simulink model "Example_2"  (R2020b)
settings: Solver=VariableStepAuto  StartTime=0.0  StopTime=0.001  RelTol=1e-3
libraries: fl_lib x10, nesl_utility x6, ee_lib x2
settings Model: Creator=zaliyazici  LastModifiedBy=zaliyazici

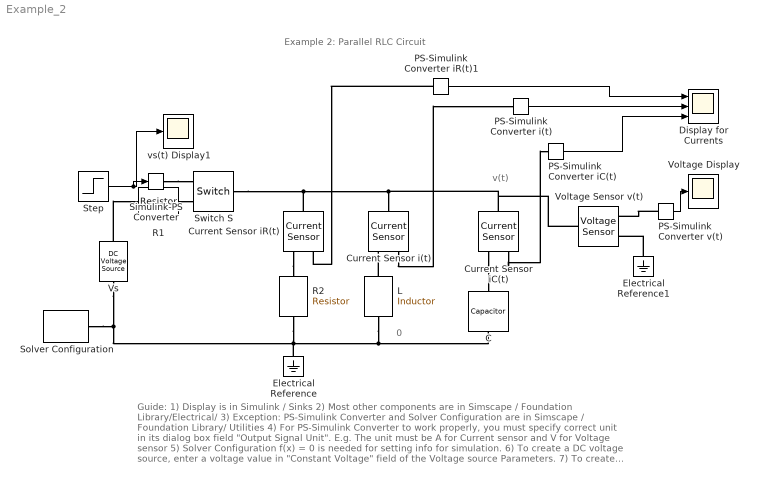
== system Example_2 ==
  note: Guide:
      | 1) Display is in Simulink / Sinks
      | 2) Most other components are in Simscape / Foundation Library/Electrical/
      | 3) Exception: PS-Simulink Converter and Solver Configuration are in Simscape / Foundation Library/ Utilities
      | 4) For PS-Simulink Converter to work properly, you must specify correct unit in its dialog box field "Output Signal Unit".
      | E.g. The unit must be A for Current sensor and V for Voltage sensor
      | 5) Solver Configuration f(x) = 0 is needed for setting info for simulation.
      | 6) To create a DC voltage source, enter a voltage value in "Constant Voltage" field of the Voltage source Parameters.
      | 7) To create "Annotation", double-click a location on project page and select "Create annotation" from the prompt. Then, type any text you want to clarify your circuit. E.g. "Display for Current".
      | 8) To understand how to use a component, right-click on the component and select "Help".
      | Measurement: Node 1 voltage $v(t)=v_C(t)=v_R(t)=V_L(t)$ , and currents $i_R(t), i_L(t)$ and $i_C(t)$
  note: Example 2: Parallel RLC Circuit
  note: 0
  note: v(t)
  C : fl_lib/Electrical/Electrical Elements/Capacitor  c=50 nF  r=1e-6 Ohm  g=0 1/Ohm  i_specify=off  i_priority=None  i=0 A  i_nominal_specify=off  i_nominal_unit=A  i_nominal_value=1  v_specify=off  v_priority=None  v=0 V  v_nominal_specify=off  v_nominal_unit=V  v_nominal_value=1  vc_specify=on  vc_priority=High  vc=5 V  vc_nominal_specify=off  vc_nominal_unit=V  vc_nominal_value=1
      settings: AttributesFormatString=|
      | %<c> %<c_unit>
      | %<vc> %<v_unit>
  Current Sensor i(t) : fl_lib/Electrical/Electrical Sensors/Current Sensor
  Current Sensor iC(t) : fl_lib/Electrical/Electrical Sensors/Current Sensor
  Current Sensor iR(t) : fl_lib/Electrical/Electrical Sensors/Current Sensor
  Display for Currents : Scope  NumInputPorts=3
  Electrical Reference : fl_lib/Electrical/Electrical Elements/Electrical Reference
  Electrical Reference1 : fl_lib/Electrical/Electrical Elements/Electrical Reference
  L : fl_lib/Electrical/Electrical Elements/Inductor  l=40 mH  r=0 Ohm  g=1e-9 1/Ohm  i_specify=off  i_priority=None  i=0 A  i_nominal_specify=off  i_nominal_unit=A  i_nominal_value=1  v_specify=off  v_priority=None  v=0 V  v_nominal_specify=off  v_nominal_unit=V  v_nominal_value=1  i_L_specify=on  i_L_priority=High  i_L=40 mA  i_L_nominal_specify=off  i_L_nominal_unit=A  i_L_nominal_value=1
      settings: AttributesFormatString=|
      | %<l> %<l_unit>
      | %<i_L> %<i_L_unit>
  PS-Simulink Converter i(t) : nesl_utility/PS-Simulink Converter  PhysicalDomain=network_engine_domain  SubClassName=ps_output  LeftPortType=input  RightPortType=output  PseudoPeriodic=off  Frequencies=[]  Unit=A  AffineConversion=off
  PS-Simulink Converter iC(t) : nesl_utility/PS-Simulink Converter  PhysicalDomain=network_engine_domain  SubClassName=ps_output  LeftPortType=input  RightPortType=output  PseudoPeriodic=off  Frequencies=[]  Unit=A  AffineConversion=off
  PS-Simulink Converter iR(t)1 : nesl_utility/PS-Simulink Converter  PhysicalDomain=network_engine_domain  SubClassName=ps_output  LeftPortType=input  RightPortType=output  PseudoPeriodic=off  Frequencies=[]  Unit=A  AffineConversion=off
  PS-Simulink Converter v(t) : nesl_utility/PS-Simulink Converter  PhysicalDomain=network_engine_domain  SubClassName=ps_output  LeftPortType=input  RightPortType=output  PseudoPeriodic=off  Frequencies=[]  Unit=V  AffineConversion=off
  R1 : ee_lib/Passive/Resistor  R=2 kOhm  R_tol=5  enable_R_tol=0  tol_distribution=1  nSigma=4  enable_operating_limits=0  operating_limit_action=2  max_working_voltage=100 V  power_rating=1 W  enable_faults=0  fault_action=1  R_faulted=inf Ohm  enable_temporal_fault=0  t_fault=1 s  enable_behavioral_fault=0  max_permissible_current=1 A  t_fail_on_current=1 s  noise_mode=0  sample_time=1e-3 s  repeatability=1  auto_seed=3439496942  user_seed=0  Tdevice=25 degC  alpha=3.93e-3 1/K  Tmeas=25 degC  thermal_mass=100 J/K  power_derating_T1=70 degC  power_derating_T2=155 degC  operating_temperature_range_vec=[-50, 150] degC  temperature_specify=off  temperature_priority=High  temperature=298.15 K  temperature_nominal_specify=off  temperature_nominal_unit=K  temperature_nominal_value=1
      settings: AttributesFormatString=%<R> %<R_unit>
  R2 : ee_lib/Passive/Resistor  R=2 kOhm  R_tol=5  enable_R_tol=0  tol_distribution=1  nSigma=4  enable_operating_limits=0  operating_limit_action=2  max_working_voltage=100 V  power_rating=1 W  enable_faults=0  fault_action=1  R_faulted=inf Ohm  enable_temporal_fault=0  t_fault=1 s  enable_behavioral_fault=0  max_permissible_current=1 A  t_fail_on_current=1 s  noise_mode=0  sample_time=1e-3 s  repeatability=1  auto_seed=2025368608  user_seed=0  Tdevice=25 degC  alpha=3.93e-3 1/K  Tmeas=25 degC  thermal_mass=100 J/K  power_derating_T1=70 degC  power_derating_T2=155 degC  operating_temperature_range_vec=[-50, 150] degC  temperature_specify=off  temperature_priority=High  temperature=298.15 K  temperature_nominal_specify=off  temperature_nominal_unit=K  temperature_nominal_value=1
      settings: AttributesFormatString=%<R> %<R_unit>
  Simulink-PS Converter : nesl_utility/Simulink-PS Converter  PhysicalDomain=network_engine_domain  SubClassName=ps_input  LeftPortType=input  RightPortType=output  PseudoPeriodic=off  Frequencies=[]  NoiseDistribution=none  NoiseParameters=[]  Unit=1  AffineConversion=off  FilteringAndDerivatives=provide  SimscapeFilterOrder=1  InputFilterTimeConstant=0.001  UdotUserProvided=0
  Solver Configuration : nesl_utility/Solver Configuration  PhysicalDomain=network_engine_domain  SubClassName=solver  LeftPortType=input  RightPortType=generic  Tones=[]  Harmonics=[]  SimulateNoise=off  Profile=off  UseLocalSampling=off  EnableSwitchedLinearOptims=on  FrequencyDomain=off  UseCCode=off  RelTol=0.001  AbsTol=1e-06  MinStep=1e-09  ToWorkspace=off  RevertToSquareIcSolve=off  NumHomotopyIterations=100  PhasorMode=off  PhasorModeNumHarmonics=1  DoDC=off  ResidualTolerance=1e-09  UseLocalSolver=off  LocalSolverChoice=NE_BACKWARD_EULER_ADVANCER  LocalSolverSampleTime=0.001  DoFixedCost=off  MaxNonlinIter=3  MaxModeIter=2  ComputeImpulses=off  ImpulseIterations=2  LinearAlgebra=auto  EquationFormulation=NE_TIME_EF  DelaysMemoryBudget=1024  AutomaticFiltering=on  FilteringTimeConstant=0.001  PartitionStorageMethod=AS_NEEDED  PartitionMemoryBudget=1024  PartitionMethod=ROBUST
  Step : Step  Time=0.0  SampleTime=0
  Switch S : fl_lib/Electrical/Electrical Elements/Switch  R_closed=0.01 Ohm  G_open=1e-8 1/Ohm  Threshold=0.5  i_specify=off  i_priority=None  i=0 A  i_nominal_specify=off  i_nominal_unit=A  i_nominal_value=1  v_specify=off  v_priority=None  v=0 V  v_nominal_specify=off  v_nominal_unit=V  v_nominal_value=1
  Voltage Display : Scope
  Voltage Sensor v(t) : fl_lib/Electrical/Electrical Sensors/Voltage Sensor
  Vs : fl_lib/Electrical/Electrical Sources/DC Voltage Source  v0=60 V
      settings: AttributesFormatString=%<v0> %<v0_unit>
  vs(t) Display1 : Scope
  wires:
  Step/1 -> vs(t) Display1/1, Simulink-PS Converter/1
  PS-Simulink Converter v(t)/1 -> Voltage Display/1
  PS-Simulink Converter iR(t)1/1 -> Display for Currents/1
  PS-Simulink Converter i(t)/1 -> Display for Currents/2
  PS-Simulink Converter iC(t)/1 -> Display for Currents/3
  connections:
  Solver Configuration/RConn1 -- Vs/RConn1 -- R2/RConn1 -- Electrical Reference/LConn1 -- L/RConn1 -- C/RConn1
  PS-Simulink Converter v(t)/LConn1 -- Voltage Sensor v(t)/RConn1
  Current Sensor iC(t)/RConn2 -- C/LConn1
  Simulink-PS Converter/RConn1 -- Switch S/RConn1
  Electrical Reference1/LConn1 -- Voltage Sensor v(t)/RConn2
  Current Sensor i(t)/RConn1 -- PS-Simulink Converter i(t)/LConn1
  L/LConn1 -- Current Sensor i(t)/RConn2
  Current Sensor iR(t)/RConn2 -- R2/LConn1
  PS-Simulink Converter iR(t)1/LConn1 -- Current Sensor iR(t)/RConn1
  Current Sensor iR(t)/LConn1 -- Voltage Sensor v(t)/LConn1 -- Current Sensor iC(t)/LConn1 -- Current Sensor i(t)/LConn1 -- Switch S/LConn1
  Current Sensor iC(t)/RConn1 -- PS-Simulink Converter iC(t)/LConn1
  R1/RConn1 -- Switch S/RConn2
  Vs/LConn1 -- R1/LConn1
